simulink model "xt6_2"  (R2014a)
settings: Solver=ode45  StartTime=0.0  StopTime=10.0  RelTol=1e-3
undefined symbols (not defined in the file or in its folder): magnitude
libraries: commanapbnd3 x1, dspstat3 x1
settings Model: Creator=tzb  LastModifiedBy=tzb

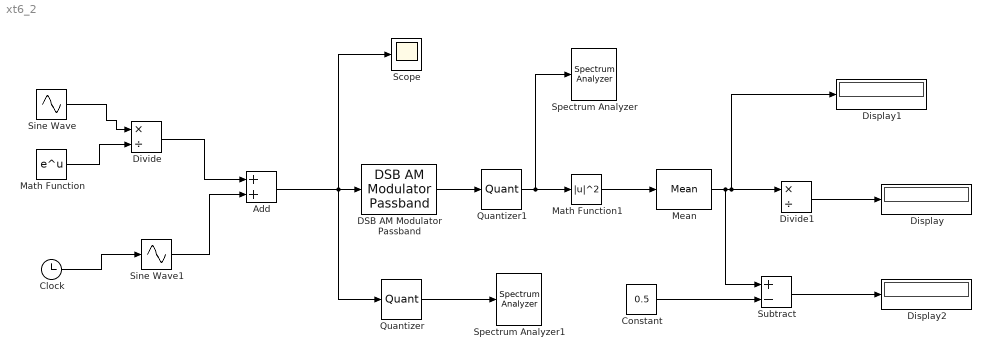
== system xt6_2 ==
  Add : Sum
  Clock : Clock
  Constant : Constant  Value=0.5
  DSB AM Modulator Passband : commanapbnd3/DSB AM Modulator Passband  Fc=300  Ph=0  Offset=1
  Display : Display
  Display1 : Display
  Display2 : Display
  Divide : Product  Inputs=*/
  Divide1 : Product  Inputs=*/
  Math Function : Math  SaturateOnIntegerOverflow=on
  Math Function1 : Math  Operator=magnitude^2  SaturateOnIntegerOverflow=on
  Mean : dspstat3/Mean  run=on  reset_popup=None  InputProcessing=Columns as channels (frame based)  directionMode=Each column  dimension=1  treatSBRowAsCol=on  roiEnable=off  roiType=Rectangles  roiPortion=Entire ROI  roiOutput=Individual statistics for each ROI  roiFlag=off  outputDataTypeStr=Inherit: Same as accumulator  outputLastDataTypeStr=Inherit: Same as accumulator  outputMin=[]  outputMax=[]  roundingMode=Floor  overflowMode=off
  Quantizer : Quantizer  QuantizationInterval=0.001  LinearizeAsGain=off  SampleTime=0.001
  Quantizer1 : Quantizer  QuantizationInterval=0.001  LinearizeAsGain=off  SampleTime=0.001
  Scope : Scope
  Sine Wave : Sin  SampleTime=0
  Sine Wave1 : Sin  SineType=Sample based  TimeSource=Use external signal  SampleTime=0
  Spectrum Analyzer : SpectrumAnalyzer
  Spectrum Analyzer1 : SpectrumAnalyzer
  Subtract : Sum  Inputs=+-
  wires:
  Clock/1 -> Sine Wave1/1
  Sine Wave1/1 -> Add/2
  Sine Wave/1 -> Divide/1
  Math Function/1 -> Divide/2
  Divide/1 -> Add/1
  Add/1 -> Quantizer/1, Scope/1, DSB AM Modulator Passband/1
  DSB AM Modulator Passband/1 -> Quantizer1/1
  Quantizer1/1 -> Spectrum Analyzer/1, Math Function1/1
  Math Function1/1 -> Mean/1
  Mean/1 -> Subtract/1, Display1/1, Divide1/1
  Divide1/1 -> Display/1
  Subtract/1 -> Display2/1
  Constant/1 -> Subtract/2
  Quantizer/1 -> Spectrum Analyzer1/1
